simulink model "pFSimulator"  (R2021a)
settings: Solver=FixedStepAuto  StartTime=0.0  StopTime=30  FixedStep=0.1  RelTol=1e-3
settings Model: Creator=jaakk  LastModifiedBy=jaakk
settings SolverCC: AlgebraicLoopSolver=TrustRegion
settings DebuggingCC: SFMachineParentedDataDiag=warning

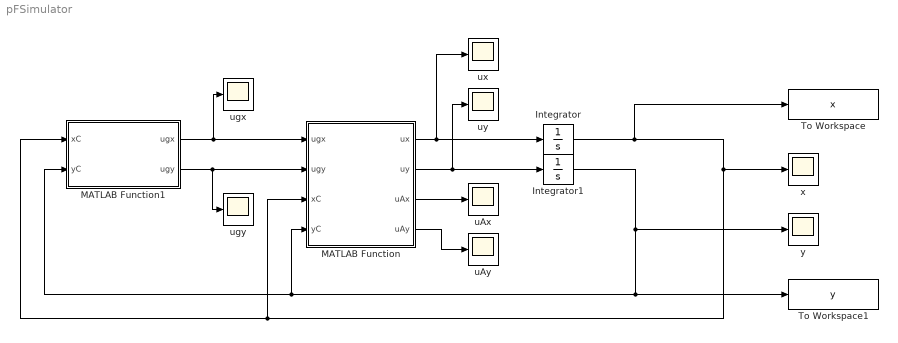
== system pFSimulator ==
  Integrator : Integrator  InitialCondition=0.17
  Integrator1 : Integrator  InitialCondition=-2.4
  MATLAB Function : MATLAB Function  TreatAsAtomicUnit=on
  MATLAB Function1 : MATLAB Function  TreatAsAtomicUnit=on
  To Workspace : ToWorkspace  VariableName=x  SaveFormat=Timeseries  SampleTime=-1
  To Workspace1 : ToWorkspace  VariableName=y  SaveFormat=Timeseries  SampleTime=-1
  uAx : Scope
  uAy : Scope
  ugx : Scope
  ugy : Scope
  ux : Scope
  uy : Scope
  x : Scope
  y : Scope
  wires:
  MATLAB Function/1(ux) -> ux/1, Integrator/1
  MATLAB Function1/1(ugx) -> ugx/1, MATLAB Function/1(ugx)
  MATLAB Function1/2(ugy) -> MATLAB Function/2(ugy), ugy/1
  MATLAB Function/2(uy) -> Integrator1/1, uy/1
  MATLAB Function/4(uAy) -> uAy/1
  MATLAB Function/3(uAx) -> uAx/1
  Integrator/1 -> MATLAB Function1/1(xC), MATLAB Function/3(xC), x/1, To Workspace/1
  Integrator1/1 -> MATLAB Function1/2(yC), MATLAB Function/4(yC), To Workspace1/1, y/1

== matlab function pFSimulator/MATLAB Function1 ==
  data: xC input; ugx output; yC input; ugy output
function [ugx, ugy]= gotogoal(xC, yC)

gx = 0;
gy = 2;
Kg = 0.05;

ugx = Kg*(2*gx - 2*xC);

ugy = Kg*(2*gy - 2*yC);

== matlab function pFSimulator/MATLAB Function ==
  data: ugx input; ugy input; ux output; xC input; yC input; uy output; uAx output; uAy output
function [ux, uy, uAx, uAy]= avoidance(ugx, ugy, xC, yC)

R = 1; % Range when avoidance is activated
r = 0.5; % Safe distance
O = [0.01 0; 0.7 0.8];
constant = 0.25; % Constant to scale u values

uAx = 0; 
uAy = 0;

h = size(O,1);

for row = 1:h
    
    obstacle = O(row,:);

    dist = sqrt((obstacle(1) - xC)^2+(obstacle(2) - yC)^2); % Distance between agent and obstacle

    if (r < dist && dist < R)
        uAxtemp = -(4*(R^2-r^2)*((dist)^2-R^2)*(xC-obstacle(1)))/(((dist)^2-r^2)^3);
        uAytemp = -(4*(R^2-r^2)*((dist)^2-R^2)*(yC-obstacle(2)))/(((dist)^2-r^2)^3);
        uAx = uAx + uAxtemp;
        uAy = uAy + uAytemp;
    end

end

u = [uAx, uAy];

if uAx ~= 0 || uAy ~= 0
    Ka = constant/sqrt(abs(uAx^2+uAy^2));
    u = Ka*u;
end

uAx = u(1);
uAy = u(2);

ux = ugx + uAx;
uy = ugy + uAy;
